simulink subsystem "rss_PhCurrHiLvl1Dia"  (R2023a)
settings: Solver=VariableStepAuto  StartTime=0.0  StopTime=10.0  RelTol=1e-3
undefined symbols (not defined in the file): Cdbl_iPhCurrMaxVal, ENM_TYPE_FALT, Gs16_iColdStrtPhCurrHiLvl1ConfTrs_C, Gs16_iColdStrtPhCurrHiLvl1RcvyTrs_C, Gs16_iPhCurrHiLvl1ConfTrs_C, Gs16_iPhCurrHiLvl1RcvyTrs_C, Gu16_ctPhCurrHiLvl1ConfCnt_C, Gu16_ctPhCurrHiLvl1RcvyCnt_C, Gu8_tColdStrtPCBTempConfTrs_C
libraries: vhit_control_library x1, lib_fault_definiteness x1
settings Model: Creator=xiaoqiang.yuan  LastModifiedBy=xiaoqiang.yuan

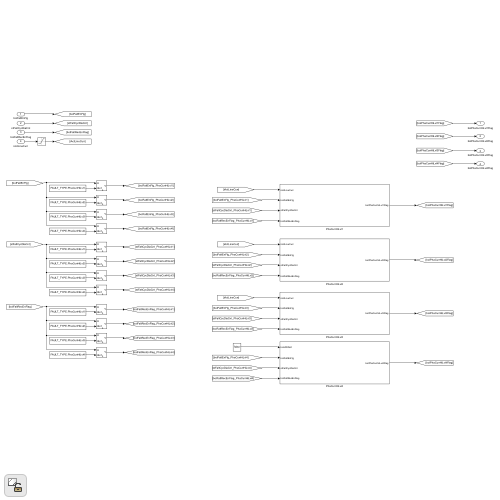
[thumbnail: Simulink's stored preview of the top-level diagram]
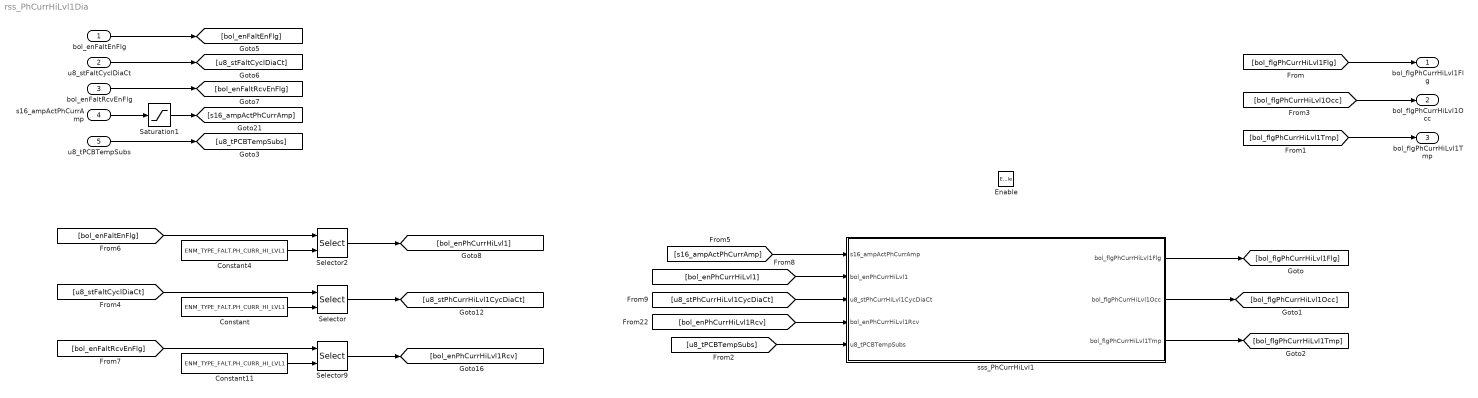
== system rss_PhCurrHiLvl1Dia ==
  bol_enFaltEnFlg : Inport  OutDataTypeStr=boolean
  u8_stFaltCyclDiaCt : Inport  Port=2  OutDataTypeStr=uint8
  bol_enFaltRcvEnFlg : Inport  Port=3  OutDataTypeStr=boolean
  s16_ampActPhCurrAmp : Inport  Port=4  OutDataTypeStr=dt_Standardize_s16p15b0
  u8_tPCBTempSubs : Inport  Port=5  OutDataTypeStr=dt_Temp_u8p0bn40
  Enable : EnablePort
  Constant : Constant  Value=ENM_TYPE_FALT.PH_CURR_HI_LVL1
  Constant11 : Constant  Value=ENM_TYPE_FALT.PH_CURR_HI_LVL1
  Constant4 : Constant  Value=ENM_TYPE_FALT.PH_CURR_HI_LVL1
  Saturation1 : Saturate  UpperLimit=Cdbl_iPhCurrMaxVal  LowerLimit=0
  Selector : Selector  IndexMode=Zero-based  InputPortWidth=Cdbl_numFaltDiaNum  IndexOptions=Index vector (port)  Indices=[1 3]  OutputSizes=1
  Selector2 : Selector  IndexMode=Zero-based  InputPortWidth=Cdbl_numFaltDiaNum  IndexOptions=Index vector (port)  Indices=[1 3]  OutputSizes=1
  Selector9 : Selector  IndexMode=Zero-based  InputPortWidth=Cdbl_numFaltDiaNum  IndexOptions=Index vector (port)  Indices=[1 3]  OutputSizes=1
  sss_PhCurrHiLvl1 : Subsystem
  bol_flgPhCurrHiLvl1Flg : Outport  OutDataTypeStr=boolean
  bol_flgPhCurrHiLvl1Occ : Outport  Port=2
  bol_flgPhCurrHiLvl1Tmp : Outport  Port=3  OutDataTypeStr=boolean
  wires:
  [bol_flgPhCurrHiLvl1Flg] -> bol_flgPhCurrHiLvl1Flg/1
  bol_enFaltEnFlg/1 -> [bol_enFaltEnFlg]
  Constant/1 -> Selector/2
  [u8_stFaltCyclDiaCt] -> Selector/1
  u8_stFaltCyclDiaCt/1 -> [u8_stFaltCyclDiaCt]
  bol_enFaltRcvEnFlg/1 -> [bol_enFaltRcvEnFlg]
  Constant4/1 -> Selector2/2
  [bol_enFaltEnFlg] -> Selector2/1
  [bol_enFaltRcvEnFlg] -> Selector9/1
  Constant11/1 -> Selector9/2
  Selector2/1 -> [bol_enPhCurrHiLvl1]
  Selector/1 -> [u8_stPhCurrHiLvl1CycDiaCt]
  Selector9/1 -> [bol_enPhCurrHiLvl1Rcv]
  [s16_ampActPhCurrAmp] -> sss_PhCurrHiLvl1/1(s16_ampActPhCurrAmp)
  [bol_enPhCurrHiLvl1] -> sss_PhCurrHiLvl1/2(bol_enPhCurrHiLvl1)
  [u8_stPhCurrHiLvl1CycDiaCt] -> sss_PhCurrHiLvl1/3(u8_stPhCurrHiLvl1CycDiaCt)
  [bol_enPhCurrHiLvl1Rcv] -> sss_PhCurrHiLvl1/4(bol_enPhCurrHiLvl1Rcv)
  sss_PhCurrHiLvl1/1(bol_flgPhCurrHiLvl1Flg) -> [bol_flgPhCurrHiLvl1Flg]
  s16_ampActPhCurrAmp/1 -> Saturation1/1
  Saturation1/1 -> [s16_ampActPhCurrAmp]
  [bol_flgPhCurrHiLvl1Occ] -> bol_flgPhCurrHiLvl1Occ/1
  sss_PhCurrHiLvl1/2(bol_flgPhCurrHiLvl1Occ) -> [bol_flgPhCurrHiLvl1Occ]
  [bol_flgPhCurrHiLvl1Tmp] -> bol_flgPhCurrHiLvl1Tmp/1
  sss_PhCurrHiLvl1/3(bol_flgPhCurrHiLvl1Tmp) -> [bol_flgPhCurrHiLvl1Tmp]
  u8_tPCBTempSubs/1 -> [u8_tPCBTempSubs]
  [u8_tPCBTempSubs] -> sss_PhCurrHiLvl1/5(u8_tPCBTempSubs)

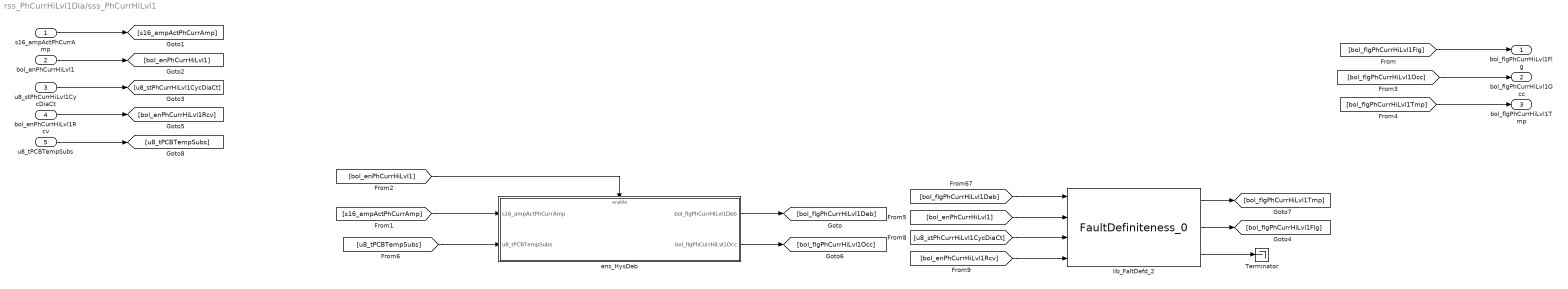
== system rss_PhCurrHiLvl1Dia/sss_PhCurrHiLvl1 ==
  s16_ampActPhCurrAmp : Inport
  bol_enPhCurrHiLvl1 : Inport  Port=2
  u8_stPhCurrHiLvl1CycDiaCt : Inport  Port=3
  bol_enPhCurrHiLvl1Rcv : Inport  Port=4
  u8_tPCBTempSubs : Inport  Port=5
  Terminator : Terminator
  ens_HysDeb : Subsystem
  lib_FaltDefd_2 : lib_fault_definiteness/FaultDefiniteness_0  lb_FaltWaitRecvCnt=Gu16_ctPhCurrHiLvl1ConfCnt_C
  bol_flgPhCurrHiLvl1Flg : Outport
  bol_flgPhCurrHiLvl1Occ : Outport  Port=2
  bol_flgPhCurrHiLvl1Tmp : Outport  Port=3
  wires:
  [u8_tPCBTempSubs] -> ens_HysDeb/2(u8_tPCBTempSubs)
  u8_tPCBTempSubs/1 -> [u8_tPCBTempSubs]
  [bol_flgPhCurrHiLvl1Tmp] -> bol_flgPhCurrHiLvl1Tmp/1
  [bol_flgPhCurrHiLvl1Occ] -> bol_flgPhCurrHiLvl1Occ/1
  ens_HysDeb/2(bol_flgPhCurrHiLvl1Occ) -> [bol_flgPhCurrHiLvl1Occ]
  lib_FaltDefd_2/1 -> [bol_flgPhCurrHiLvl1Tmp]
  lib_FaltDefd_2/2 -> [bol_flgPhCurrHiLvl1Flg]
  lib_FaltDefd_2/3 -> Terminator/1
  [bol_enPhCurrHiLvl1] -> ens_HysDeb/Enable
  [s16_ampActPhCurrAmp] -> ens_HysDeb/1(s16_ampActPhCurrAmp)
  ens_HysDeb/1(bol_flgPhCurrHiLvl1Deb) -> [bol_flgPhCurrHiLvl1Deb]
  bol_enPhCurrHiLvl1Rcv/1 -> [bol_enPhCurrHiLvl1Rcv]
  u8_stPhCurrHiLvl1CycDiaCt/1 -> [u8_stPhCurrHiLvl1CycDiaCt]
  bol_enPhCurrHiLvl1/1 -> [bol_enPhCurrHiLvl1]
  [bol_flgPhCurrHiLvl1Flg] -> bol_flgPhCurrHiLvl1Flg/1
  s16_ampActPhCurrAmp/1 -> [s16_ampActPhCurrAmp]
  [bol_enPhCurrHiLvl1Rcv] -> lib_FaltDefd_2/4
  [u8_stPhCurrHiLvl1CycDiaCt] -> lib_FaltDefd_2/3
  [bol_enPhCurrHiLvl1] -> lib_FaltDefd_2/2
  [bol_flgPhCurrHiLvl1Deb] -> lib_FaltDefd_2/1

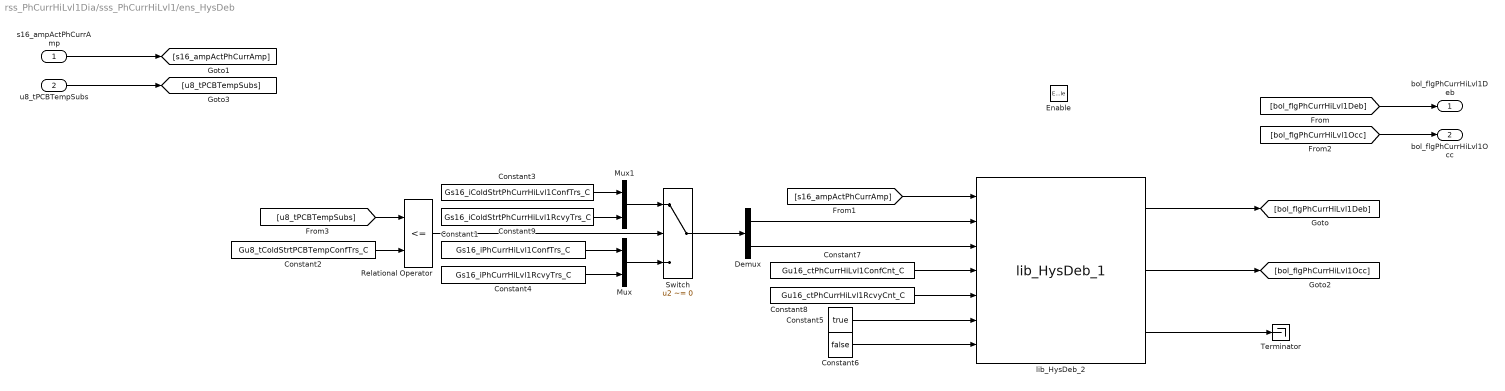
== system rss_PhCurrHiLvl1Dia/sss_PhCurrHiLvl1/ens_HysDeb ==
  s16_ampActPhCurrAmp : Inport
  u8_tPCBTempSubs : Inport  Port=2
  Enable : EnablePort
  Constant1 : Constant  Value=Gs16_iPhCurrHiLvl1ConfTrs_C
  Constant2 : Constant  Value=Gu8_tColdStrtPCBTempConfTrs_C
  Constant3 : Constant  Value=Gs16_iColdStrtPhCurrHiLvl1ConfTrs_C
  Constant4 : Constant  Value=Gs16_iPhCurrHiLvl1RcvyTrs_C
  Constant5 : Constant  Value=true  OutDataTypeStr=boolean
  Constant6 : Constant  Value=false  OutDataTypeStr=boolean
  Constant7 : Constant  Value=Gu16_ctPhCurrHiLvl1ConfCnt_C
  Constant8 : Constant  Value=Gu16_ctPhCurrHiLvl1RcvyCnt_C
  Constant9 : Constant  Value=Gs16_iColdStrtPhCurrHiLvl1RcvyTrs_C
  Demux : Demux  Outputs=2
  Mux : Mux  Inputs=2
  Mux1 : Mux  Inputs=2
  Relational Operator : RelationalOperator  Operator=<=  OutDataTypeStr=boolean  RndMeth=Simplest  InputSameDT=off
  Switch : Switch  Criteria=u2 ~= 0  SaturateOnIntegerOverflow=off  InputSameDT=off
  Terminator : Terminator
  lib_HysDeb_2 : vhit_control_library/lib_HysDeb_1  lb_parInitOutp=0
  bol_flgPhCurrHiLvl1Deb : Outport
  bol_flgPhCurrHiLvl1Occ : Outport  Port=2
  wires:
  Switch/1 -> Demux/1
  Demux/2 -> lib_HysDeb_2/3
  Demux/1 -> lib_HysDeb_2/2
  Mux1/1 -> Switch/1
  Constant3/1 -> Mux1/1
  Constant9/1 -> Mux1/2
  Mux/1 -> Switch/3
  Constant4/1 -> Mux/2
  Constant1/1 -> Mux/1
  Relational Operator/1 -> Switch/2
  [u8_tPCBTempSubs] -> Relational Operator/1
  Constant2/1 -> Relational Operator/2
  u8_tPCBTempSubs/1 -> [u8_tPCBTempSubs]
  [bol_flgPhCurrHiLvl1Occ] -> bol_flgPhCurrHiLvl1Occ/1
  lib_HysDeb_2/3 -> Terminator/1
  lib_HysDeb_2/2 -> [bol_flgPhCurrHiLvl1Occ]
  lib_HysDeb_2/1 -> [bol_flgPhCurrHiLvl1Deb]
  Constant8/1 -> lib_HysDeb_2/5
  Constant7/1 -> lib_HysDeb_2/4
  Constant6/1 -> lib_HysDeb_2/7
  Constant5/1 -> lib_HysDeb_2/6
  [s16_ampActPhCurrAmp] -> lib_HysDeb_2/1
  s16_ampActPhCurrAmp/1 -> [s16_ampActPhCurrAmp]
  [bol_flgPhCurrHiLvl1Deb] -> bol_flgPhCurrHiLvl1Deb/1
